simulink model "MotionController"  (R2020b)
settings: Solver=VariableStepAuto  StartTime=0.0  StopTime=10.0  RelTol=1e-3
values from neighbouring files (symbols this model uses):
  lqgController = -0.76499999999998936 -0.64280114808522471 -0.33035598888106893 -0.10979041252358804    [VehicleModelDictionary.sldd]
  ltiSys = ss(ltiSys.A, ltiSys.B, C, D)    [ControllerDesign.m]    (also in LinearAnalysis.m = ss(A, B, C, D); VehicleModelDictionary.sldd = 4.0 2.0
                22.0
                
              )
  MotorParameters = 34.0    [VehicleModelDictionary.sldd]    (also in VehicleParametersDictionary.sldd)
settings Model: Creator=Gonzalo Fernández  LastModifiedBy=Gonzalo Fernández

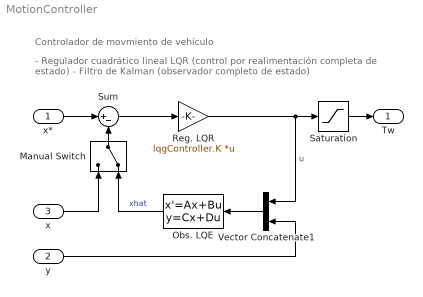
== system MotionController ==
  note: - Regulador cuadrático lineal LQR (control por realimentación completa de estado)
      | - Filtro de Kalman (observador completo de estado)
  note: Controlador de movmiento de vehículo
  x* : Inport  PortDimensions=[4, 1]
  y : Inport  Port=2  PortDimensions=[3, 1]
  x : Inport  Port=3  PortDimensions=[4, 1]
  Manual Switch : ManualSwitch  CurrentSetting=0
  Obs. LQE : StateSpace  A=ltiSys.A-lqgController.L*ltiSys.C  B=[ltiSys.B(:, 1), lqgController.L]  C=eye(4)  D=zeros(4, size([ltiSys.B(:, 1), lqgController.L], 2))  InitialCondition=0
  Reg. LQR : Gain  Gain=lqgController.K  Multiplication=Matrix(K*u)
  Saturation : Saturate  UpperLimit=2*MotorParameters.maxTorque  LowerLimit=-2*MotorParameters.maxTorque  LinearizeAsGain=off
  Sum : Sum  Inputs=|+-
  Vector Concatenate1 : Concatenate
  Tw : Outport
  wires:
  x*/1 -> Sum/1
  Sum/1 -> Reg. LQR/1
  Reg. LQR/1 -> Saturation/1, Vector Concatenate1/1  "u"
  Obs. LQE/1 -> Manual Switch/2  "xhat"
  Vector Concatenate1/1 -> Obs. LQE/1
  y/1 -> Vector Concatenate1/2
  x/1 -> Manual Switch/1
  Manual Switch/1 -> Sum/2
  Saturation/1 -> Tw/1
